simulink model "spatiul_starilor_2"  (R2020a)
settings: Solver=VariableStepAuto  StartTime=0.0  StopTime=3  RelTol=1e-3
undefined symbols (not defined in the file): F, J, kt, L, R, U
settings Model: Creator=adrian.negoita1804  LastModifiedBy=adrian.negoita1804

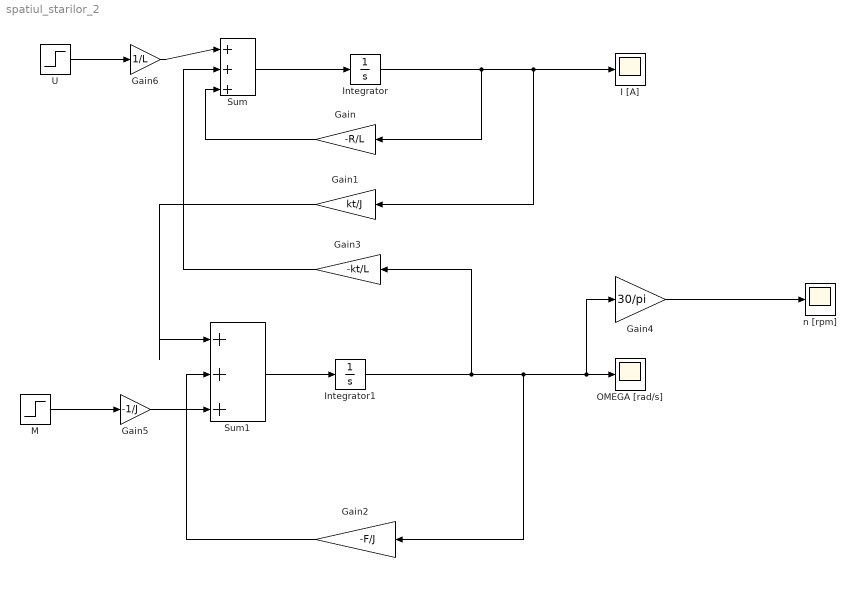
== system spatiul_starilor_2 ==
  Gain : Gain  Gain=-R/L
  Gain1 : Gain  Gain=kt/J
  Gain2 : Gain  Gain=-F/J
  Gain3 : Gain  Gain=-kt/L
  Gain4 : Gain  Gain=30/pi
  Gain5 : Gain  Gain=-1/J
  Gain6 : Gain  Gain=1/L
  I [A] : Scope
  Integrator : Integrator
  Integrator1 : Integrator
  M : Step  After=12  SampleTime=0
  OMEGA [rad/s] : Scope
  Sum : Sum  Inputs=|+++
  Sum1 : Sum  Inputs=|+++
  U : Step  Time=0  After=U  SampleTime=0
  n [rpm] : Scope
  wires:
  U/1 -> Gain6/1
  M/1 -> Gain5/1
  Gain6/1 -> Sum/1
  Sum/1 -> Integrator/1
  Gain5/1 -> Sum1/3
  Sum1/1 -> Integrator1/1
  Gain2/1 -> Sum1/2
  Integrator/1 -> Gain/1, Gain1/1, I [A]/1
  Gain/1 -> Sum/3
  Gain3/1 -> Sum/2
  Gain1/1 -> Sum1/1
  Integrator1/1 -> Gain3/1, Gain2/1, Gain4/1, OMEGA [rad/s]/1
  Gain4/1 -> n [rpm]/1
